simulink model "lin_2in_3d"  (Simulink 7.9)
settings: Solver=ode45  StartTime=0.0  StopTime=tend  FixedStep=params.th  MaxStep=0.01  RelTol=1e-6  AbsTol=1e-3
settings Model: Creator=puri  LastModifiedBy=Manu
settings CodeAppCC: CustomSymbolStrType=$N$R$M_T
settings GRTTargetCC: CodeReplacementLibrary=None  CPPClassGenCompliant=on

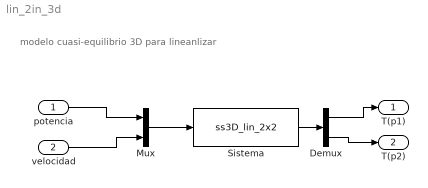
== system lin_2in_3d ==
  note: modelo cuasi-equilibrio 3D para lineanlizar
  potencia : Inport
  velocidad : Inport  Port=2
  Demux : Demux  Outputs=2
  Mux : Mux  Inputs=2
  Sistema : S-Function  FunctionName=ss3D_lin_2x2  EnableBusSupport=off
      settings: DeleteFcn=shh = get(0,'ShowHiddenHandles');set(0,'ShowHiddenHandles','on');if ~isempty(findobj('type','figure','name','dblcart1 Animation'));close('dblcart1 Animation'); end;set(0,'ShowHiddenHandles',shh);
  T(p1) : Outport
  T(p2) : Outport  Port=2
  wires:
  Mux/1 -> Sistema/1
  potencia/1 -> Mux/1
  velocidad/1 -> Mux/2
  Sistema/1 -> Demux/1
  Demux/1 -> T(p1)/1
  Demux/2 -> T(p2)/1
